simulink model "Lab_6"  (R2022b)
settings: Solver=VariableStepAuto  StartTime=0.0  StopTime=10.0  RelTol=1e-3
libraries: simulink x1
settings Model: Creator=Azlaan  LastModifiedBy=Azlaan

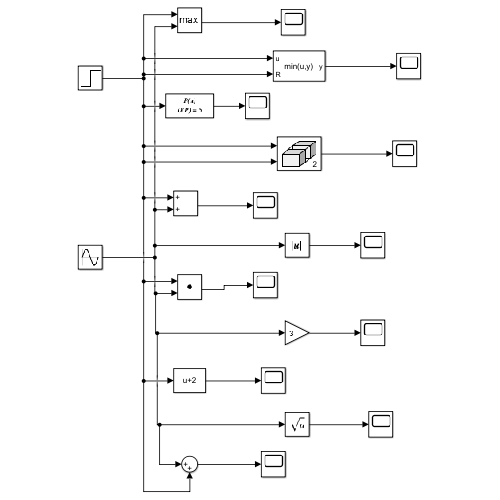
[thumbnail: Simulink's stored preview of the top-level diagram]
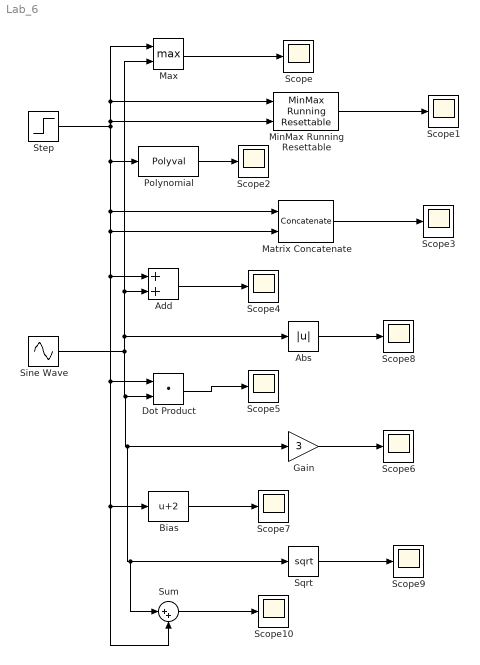
== system Lab_6 ==
  Abs : Abs  SaturateOnIntegerOverflow=off
  Add : Sum
  Bias : Bias  Bias=2  SaturateOnIntegerOverflow=off
  Dot Product : DotProduct  OutDataTypeStr=Inherit: Inherit via internal rule
  Gain : Gain  Gain=3
  Matrix Concatenate : Concatenate  Mode=Multidimensional array  ConcatenateDimension=2
  Max : MinMax  Function=max  Inputs=2
  MinMax Running Resettable : simulink/Math Operations/MinMax Running Resettable  Function=min  vinit=0.0
  Polynomial : Polyval  Coefs=[ +2.081618890e-019, -1.441693666e-014, +4.719686976e-010, -8.536869453e-006, +1.621573104e-001, -8.087801117e+001 ]
  Scope{,1..10} (11 alike) : Scope
  Sine Wave : Sin  SampleTime=0
  Sqrt : Sqrt  OutputSignalType=complex
  Step : Step  SampleTime=0
  Sum : Sum  Inputs=|++
  wires:
  Max/1 -> Scope/1
  Step/1 -> MinMax Running Resettable/1, Max/1, MinMax Running Resettable/2, Matrix Concatenate/1, Sum/2, Bias/1, Dot Product/1, Add/1, Matrix Concatenate/2, Polynomial/1
  MinMax Running Resettable/1 -> Scope1/1
  Polynomial/1 -> Scope2/1
  Matrix Concatenate/1 -> Scope3/1
  Add/1 -> Scope4/1
  Dot Product/1 -> Scope5/1
  Gain/1 -> Scope6/1
  Bias/1 -> Scope7/1
  Sine Wave/1 -> Sum/1, Sqrt/1, Gain/1, Dot Product/2, Abs/1, Add/2, Max/2
  Abs/1 -> Scope8/1
  Sqrt/1 -> Scope9/1
  Sum/1 -> Scope10/1
